simulink model "practice_4_model"  (R2021b)
settings: Solver=VariableStepAuto  StartTime=0.0  StopTime=15  RelTol=1e-3
values from neighbouring files (symbols this model uses):
  a11 = -0.159    [lab_4.m]    (also in practice_4.m; practice_4_script.m = -0.1253; praktika.m)
  a12 = 0.267    [lab_4.m]    (also in practice_4.m; practice_4_script.m = -0.004637; praktika.m)
  b = -0.002198    [practice_4_script.m]
  k1 = 10    [practice_4.m]    (also in practice_4_script.m; praktika.m)
  k2 = 20    [practice_4.m]    (also in practice_4_script.m = 1; praktika.m)
  k3 = 5    [practice_4.m]    (also in practice_4_script.m = -0.2; praktika.m)
libraries: checkpacklib x1
settings Model: Creator=vkad  LastModifiedBy=vkad

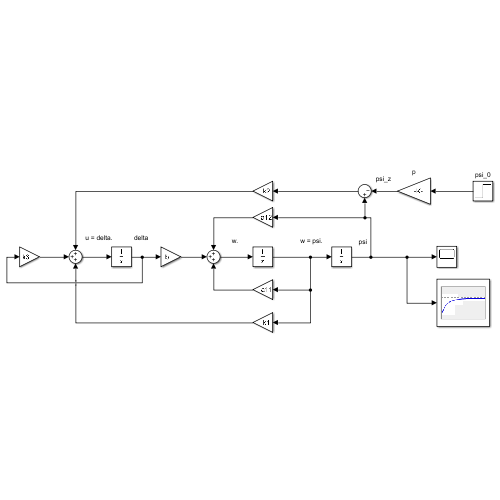
[thumbnail: Simulink's stored preview of the top-level diagram]
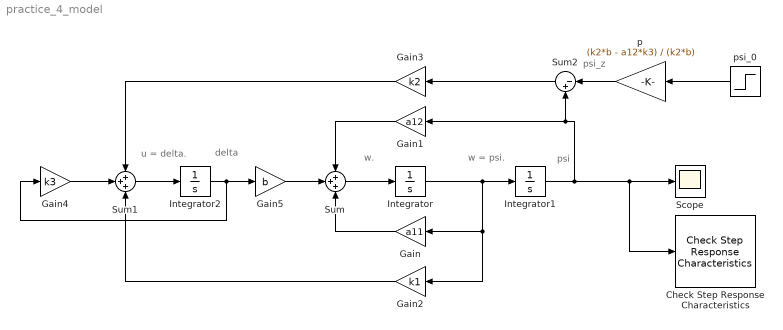
== system practice_4_model ==
  note: psi_z
  note: delta
  note: psi
  note: u = delta.
  note: w = psi.
  note: w.
  Check Step Response Characteristics : checkpacklib/Check Step Response  Characteristics  InstantiateOnLoad=on  enabled=on  stopWhenAssertionFail=off  export=off  ViewDlgPos=[]  OpenViewOnLoad=off  LaunchViewOnOpen=off  TimeUnits=seconds  EnableStepResponseBound=on  InitialValue=0  FinalValue=1  StepTime=0  RiseTime=5  PercentRise=80  SettlingTime=7  PercentSettling=1  PercentOvershoot=10  PercentUndershoot=1
      settings: SourceProductBaseCode=CT,ID,MT,SO
  Gain : Gain  Gain=a11
  Gain1 : Gain  Gain=a12
  Gain2 : Gain  Gain=k1
  Gain3 : Gain  Gain=k2
  Gain4 : Gain  Gain=k3
  Gain5 : Gain  Gain=b
  Integrator : Integrator
  Integrator1 : Integrator
  Integrator2 : Integrator
  Scope : Scope
  Sum : Sum  Inputs=+++
  Sum1 : Sum  Inputs=+++
  Sum2 : Sum  Inputs=|-+
  p : Gain  Gain=(k2*b - a12*k3) / (k2*b)
  psi_0 : Step  Time=0  SampleTime=0
  wires:
  Integrator/1 -> Integrator1/1, Gain/1, Gain2/1
  Sum/1 -> Integrator/1
  Gain/1 -> Sum/3
  Integrator1/1 -> Check Step Response Characteristics/1, Scope/1, Sum2/2, Gain1/1
  Gain1/1 -> Sum/1
  Integrator2/1 -> Gain5/1, Gain4/1
  Sum1/1 -> Integrator2/1
  Gain2/1 -> Sum1/3
  Sum2/1 -> Gain3/1
  Gain3/1 -> Sum1/1
  Gain4/1 -> Sum1/2
  Gain5/1 -> Sum/2
  p/1 -> Sum2/1
  psi_0/1 -> p/1
